simulink model "kongzhiqi2_nijunkang"  (R2019b)
settings: Solver=ode4  StartTime=0.0  StopTime=10  FixedStep=0.001  RelTol=1e-3  EnableMultiTasking=on
settings Model: PauseTimes=0.2  Creator=84360  LastModifiedBy=user
settings DataIOCC: ReturnWorkspaceOutputs=off
settings OptimizationCC: LifeSpan=inf
settings DebuggingCC: SFUnexpectedBacktrackingDiag=warning  SFNoUnconditionalDefaultTransitionDiag=warning  ArithmeticOperatorsInVariantConditions=warning
settings SFSimCC: SimUseLocalCustomCode=off  CustomCodeUndefinedFunction=UseInterfaceOnly
settings RTWCC: RTWUseLocalCustomCode=off
settings CodeAppCC: StateflowObjectComments=on
settings GRTTargetCC: TargetLangStandard=C89/C90 (ANSI)  GeneratePreprocessorConditionals=Disable all
settings ConfigComp: CovMetricSettings=dw  CovHtmlReporting=on  CovSaveCumulativeToWorkspaceVar=on  CovSaveSingleToWorkspaceVar=on  CovExternalEMLEnable=off

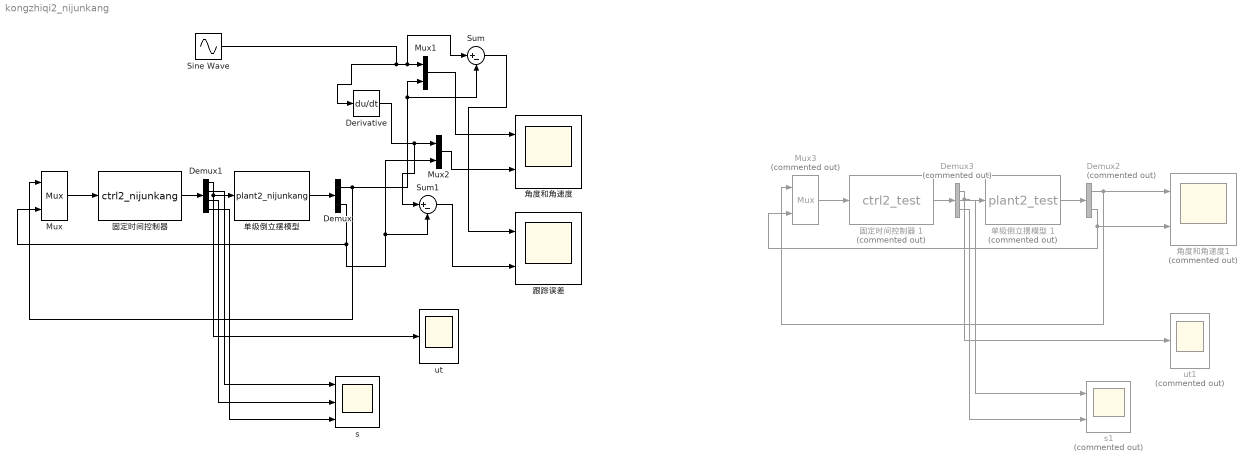
== system kongzhiqi2_nijunkang ==
  Demux : Demux  Outputs=2
  Demux1 : Demux
  Demux2 : Demux  Commented=on  Outputs=2
  Demux3 : Demux  Commented=on  Outputs=3
  Derivative : Derivative
  Mux : Mux  Inputs=2
  Mux1 : Mux  Inputs=2
  Mux2 : Mux  Inputs=2
  Mux3 : Mux  Commented=on  Inputs=2
  Sine Wave : Sin  Frequency=1/2  SampleTime=0
  Sum : Sum  Inputs=|+-
  Sum1 : Sum  Inputs=|+-
  s : Scope  NumInputPorts=3
  s1 : Scope  Commented=on  NumInputPorts=2
  ut : Scope
  ut1 : Scope  Commented=on
  "单级倒立摆模型 " : S-Function  FunctionName=plant2_nijunkang  SFunctionDeploymentMode=off  EnableBusSupport=off
  单级倒立摆模型 1 : S-Function  Commented=on  FunctionName=plant2_test  SFunctionDeploymentMode=off  EnableBusSupport=off
  "固定时间控制器 " : S-Function  FunctionName=ctrl2_nijunkang  SFunctionDeploymentMode=off  EnableBusSupport=off
  固定时间控制器 1 : S-Function  Commented=on  FunctionName=ctrl2_test  SFunctionDeploymentMode=off  EnableBusSupport=off
  角度和角速度 : Scope  NumInputPorts=2
  角度和角速度1 : Scope  Commented=on  NumInputPorts=2
  跟踪误差 : Scope  NumInputPorts=2
  wires:
  Demux/1 -> Mux1/2, Sum/2, Mux/1
  Demux1/1 -> "单级倒立摆模型 "/1, ut/1
  Demux/2 -> Mux/2, Sum1/2, Mux2/2
  Demux1/2 -> s/1
  Mux1/1 -> 角度和角速度/1
  Mux2/1 -> 角度和角速度/2
  Derivative/1 -> Sum1/1, Mux2/1
  Sine Wave/1 -> Derivative/1, Sum/1, Mux1/1
  Mux/1 -> "固定时间控制器 "/1
  "固定时间控制器 "/1 -> Demux1/1
  "单级倒立摆模型 "/1 -> Demux/1
  Demux2/2 -> Mux3/2, 角度和角速度1/2
  Demux3/2 -> s1/1
  Demux3/1 -> 单级倒立摆模型 1/1, ut1/1
  Mux3/1 -> 固定时间控制器 1/1
  固定时间控制器 1/1 -> Demux3/1
  Demux2/1 -> Mux3/1, 角度和角速度1/1
  单级倒立摆模型 1/1 -> Demux2/1
  Demux3/3 -> s1/2
  Demux1/3 -> s/2
  Sum/1 -> 跟踪误差/1
  Sum1/1 -> 跟踪误差/2
  Demux1/4 -> s/3
